simulink model "Junctions9"  (Simulink 5.0)
settings: Solver=FixedStepDiscrete  StartTime=0.0  StopTime=10.0  RelTol=1e-3
settings Model: Creator=sofronis  LastModifiedBy=scaife  ExtModeAutoUpdateStatusClock=off  AlgebraicLoopMsg=error

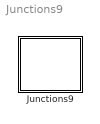
== system Junctions9 ==
  Junctions9 : Stateflow chart

== stateflow chart Junctions9 ==
  state A
  state C
  state B
  A -> (junction 6) : [true] {a+=1}
  (junction 6) -> (junction 7) : [true] {a+=10}
  (junction 7) -> B : [false] {a+=100}
  (default) -> A : {a = 0}
  (junction 6) -> C : [true] {a+=1000}
  data: true constant =1; a local; false constant
